simulink model "signalcontainer_th"  (R2018b)
settings: Solver=VariableStepAuto  StartTime=0.0  StopTime=10.0  RelTol=1e-3
settings Model: Creator=mitch  LastModifiedBy=mcobb

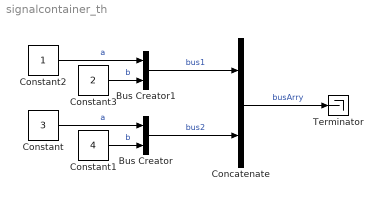
== system signalcontainer_th ==
  Bus Creator : BusCreator  Inputs=2  OutDataTypeStr=Bus: sldemo_bus_arrays_busobject  NonVirtualBus=on
  Bus Creator1 : BusCreator  Inputs=2  OutDataTypeStr=Bus: sldemo_bus_arrays_busobject  NonVirtualBus=on
  Concatenate : Concatenate
  Constant : Constant  Value=3
  Constant1 : Constant  Value=4
  Constant2 : Constant
  Constant3 : Constant  Value=2
  Terminator : Terminator
  wires:
  Bus Creator/1 -> Concatenate/2  "bus2"
  Bus Creator1/1 -> Concatenate/1  "bus1"
  Constant3/1 -> Bus Creator1/2  "b"
  Constant2/1 -> Bus Creator1/1  "a"
  Constant/1 -> Bus Creator/1  "a"
  Constant1/1 -> Bus Creator/2  "b"
  Concatenate/1 -> Terminator/1  "busArry"
